simulink model "Q2_ViralPanchal"  (R2021a)
settings: Solver=VariableStepAuto  StartTime=0.0  StopTime=8  RelTol=1e-3
undefined symbols (not defined in the file): sigbuilder_block
settings Model: Creator=viral  LastModifiedBy=viral

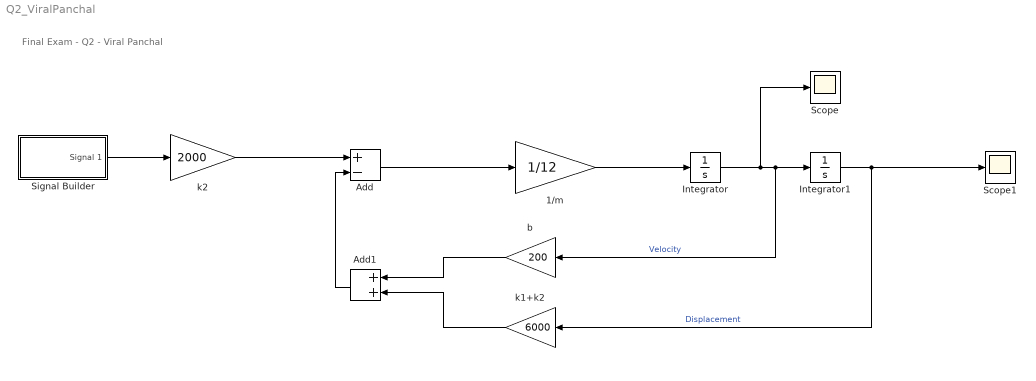
== system Q2_ViralPanchal ==
  note: Final Exam - Q2 - Viral Panchal
  1/m : Gain  Gain=1/12
  Add : Sum  Inputs=+-
  Add1 : Sum
  Integrator : Integrator
  Integrator1 : Integrator
  Scope : Scope
  Scope1 : Scope
  Signal Builder : Subsystem  Tag=STV Subsys  LoadFcn=sigbuilder_block('load');  StartFcn=sigbuilder_block('start');  StopFcn=sigbuilder_block('stop');  ClipboardFcn=sigbuilder_block('clipboard');  mask(Sigbuilder block){tuvar=[0:10]}
      mask help: Simulink:masks:SigbuilderBlock_MD
      mask init:
      | if ~strcmp(get_param(bdroot(gcbh),'SimulationStatus'),'stopped') tuvar = sigbuilder_block('maskInit'); end
      settings: CopyFcn=sigbuilder_block('copy');  DeleteFcn=sigbuilder_block('delete');  ModelCloseFcn=sigbuilder_block('modelClose');  PreSaveFcn=sigbuilder_block('preSave');  PauseFcn=sigbuilder_block('pause');  ContinueFcn=sigbuilder_block('continue');  NameChangeFcn=sigbuilder_block('namechange');  OpenFcn=sigbuilder_block('open',[402 127.2 550.8 400.2 ]);  CloseFcn=sigbuilder_block('close');
      mask Display: plot(0, 0, 100, 100,[2, 2, 32, 32, 2], [68, 8, 8, 68, 68],[32, 2], [38, 38], [32, 19, 2],[53, 60, 44], [32, 17, 17, 2],[16, 16, 31, 31]);txt = getActiveGroup(gcbh);text(2, 100, txt,'verticalAlignment', 'top');
  b : Gain  Gain=200
  k1+k2 : Gain  Gain=6000
  k2 : Gain  Gain=2000
  wires:
  k2/1 -> Add/1
  Add1/1 -> Add/2
  b/1 -> Add1/1
  k1+k2/1 -> Add1/2
  Add/1 -> 1/m/1
  1/m/1 -> Integrator/1
  Integrator/1 -> Scope/1, b/1, Integrator1/1  "Velocity"
  Integrator1/1 -> k1+k2/1, Scope1/1  "Displacement"
  Signal Builder/1(Signal 1) -> k2/1

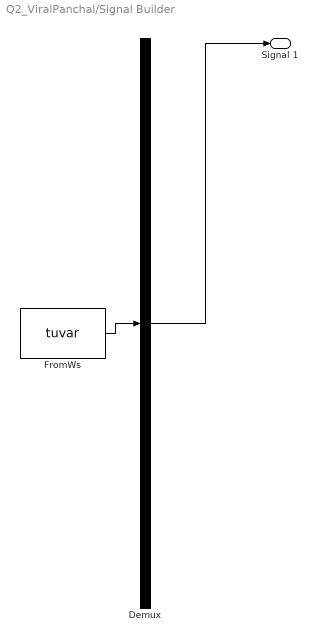
== system Q2_ViralPanchal/Signal Builder ==
  Demux : Demux  Tag=STV Demux  Outputs=1
      settings: DisplayOption=none
  FromWs : FromWorkspace  Tag=STV FromWs  VariableName=tuvar
      SigBuilderData=|
      | common.afterFinalStr = 'Extrapolate'
      | common.sampleTime = 0
      | dataSet.timeRange = [0 10]
      | dataSet.name = 'Group 1'
      | sbobj.Groups.Name = 'Group 1'
      | sbobj.Groups.Signals.Name = 'Signal 1'
      | sbobj.Groups.Signals.XData = [0 1.5 2 3.5 4 5.5 6 10]
      | sbobj.Groups.Signals.YData = [0 0.03 0 0.03 0 0.03 0 -0.0064]
  Signal 1 : Outport  Tag=STV Outport
  wires:
  Demux/1 -> Signal 1/1
  FromWs/1 -> Demux/1
